simulink model "KF_Problem5"  (R2025b)
settings: Solver=FixedStepDiscrete  StartTime=0.0  StopTime=34  FixedStep=1  RelTol=1e-3
libraries: matrix_library x3, simulink x2
settings Model: Creator=xox  LastModifiedBy=xox
settings OptimizationCC: BlockReduction=off  DefaultParameterBehavior=Inlined  BufferReuse=off

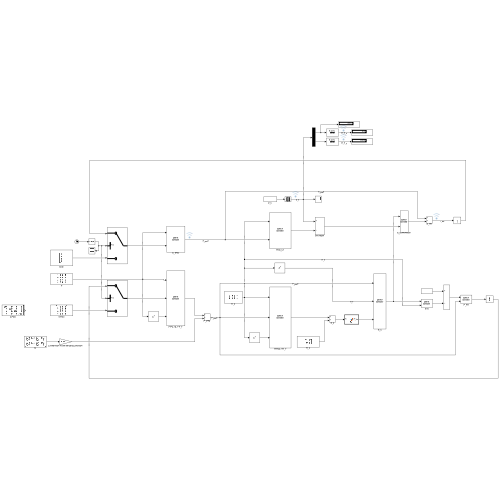
[thumbnail: Simulink's stored preview of the top-level diagram]
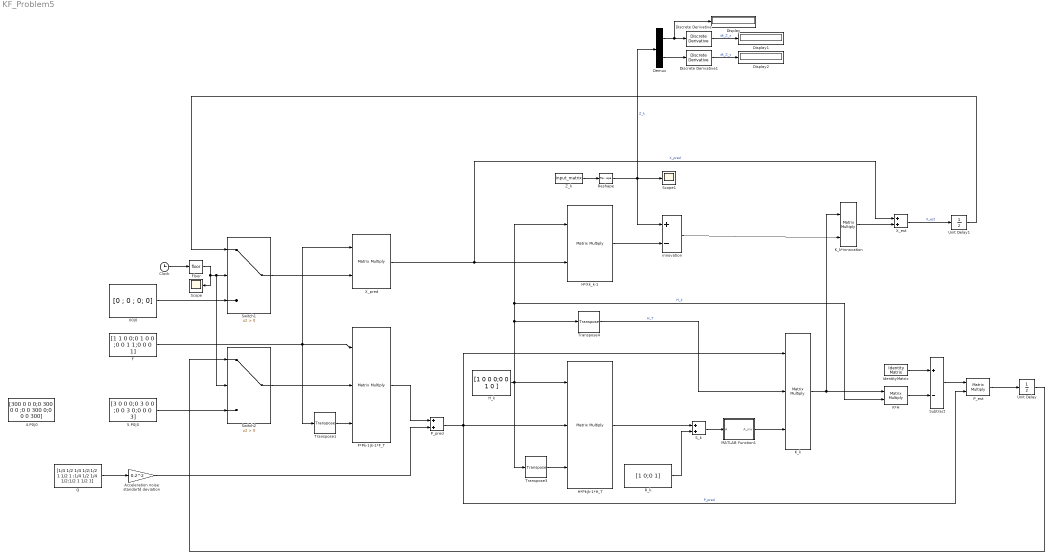
== system KF_Problem5 ==
  4.P0|0 : Constant  Value=[300 0 0 0;0 300 0 0 ;0 0 300 0;0 0 0 300]  VectorParams1D=off
  5.P0|0 : Constant  Value=[3 0 0 0;0 3 0 0 ;0 0 3 0;0 0 0 3]  VectorParams1D=off
  Acceleration noise standartd deviation : Gain  Gain=0.2^2
  Clock : Clock
  Demux : Demux  Outputs=2
  Discrete Derivative : simulink/Discrete/Discrete Derivative  gainval=1.0  ICPrevScaledInput=0.0  OutMin=[]  OutMax=[]  OutDataType=fixdt(1, 16)  OutScaling=2^-10  DoSatur=off
  Discrete Derivative1 : simulink/Discrete/Discrete Derivative  gainval=1.0  ICPrevScaledInput=0.0  OutMin=[]  OutMax=[]  OutDataType=fixdt(1, 16)  OutScaling=2^-10  DoSatur=off
  Display : Display
  Display1 : Display
  Display2 : Display
  F : Constant  Value=[1 1 0 0;0 1 0 0 ;0 0 1 1;0 0 0 1]  VectorParams1D=off
  F*Pk-1|k-1*F_T : Product  Inputs=3  Multiplication=Matrix(*)
  Floor : Rounding
  H*Pk|k-1*H_T : Product  Inputs=3  Multiplication=Matrix(*)
  H*Xk_k-1 : Product  Multiplication=Matrix(*)
  H_k : Constant  Value=[1 0 0 0;0 0 1 0 ]  VectorParams1D=off
  IdentityMatrix : IdentityMatrix  OutputDimensions=4
  K*H : Product  Multiplication=Matrix(*)
  K_k : Product  Inputs=3  Multiplication=Matrix(*)
  K_k*innovation : Product  Multiplication=Matrix(*)
  MATLAB Function1 : MATLAB Function  TreatAsAtomicUnit=on
  P_est : Product  Multiplication=Matrix(*)
  P_pred : Sum
  Q : Constant  Value=[1/4 1/2 1/4 1/2;1/2 1 1/2 1 ;1/4 1/2 1/4 1/2;1/2 1 1/2 1]  VectorParams1D=off
  R_k : Constant  Value=[1 0;0 1]  VectorParams1D=off
  Reshape : Reshape  OutputDimensionality=Column vector (2-D)
  S_k : Sum
  Scope : Scope
      settings: ActiveDisplayYMinimum=-7.79614286700194  ActiveDisplayYMaximum=47.001324962719174
  Scope1 : Scope
      settings: ActiveDisplayYMinimum=-433.90733679932936  ActiveDisplayYMaximum=356.88208874930586
  Subtract : Sum  Inputs=+-
  Switch1 : Switch  Criteria=u2 > Threshold  SaturateOnIntegerOverflow=off  InputSameDT=off
  Switch2 : Switch  Criteria=u2 > Threshold  SaturateOnIntegerOverflow=off  InputSameDT=off
  Transpose1 : matrix_library/Transpose
  Transpose3 : matrix_library/Transpose
  Transpose4 : matrix_library/Transpose
  Unit Delay : UnitDelay  SampleTime=-1  HasFrameUpgradeWarning=on
  Unit Delay1 : UnitDelay  SampleTime=-1  HasFrameUpgradeWarning=on
  X0|0 : Constant  Value=[0 ; 0 ; 0; 0]  VectorParams1D=off
  X_est : Sum
  X_pred : Product  Multiplication=Matrix(*)
  Z_k : FromWorkspace  VariableName=input_matrix
  innovation : Sum  Inputs=+-
  wires:
  Q/1 -> Acceleration noise standartd deviation/1
  S_k/1 -> MATLAB Function1/1(A)
  Clock/1 -> Floor/1
  Floor/1 -> Scope/1, Switch2/2, Switch1/2
  X0|0/1 -> Switch1/3
  F/1 -> Transpose1/1, F*Pk-1|k-1*F_T/1, X_pred/1
  Switch1/1 -> X_pred/2
  X_pred/1 -> X_est/1, H*Xk_k-1/2  "X_pred"
  Switch2/1 -> F*Pk-1|k-1*F_T/2
  Transpose1/1 -> F*Pk-1|k-1*F_T/3
  F*Pk-1|k-1*F_T/1 -> P_pred/1
  Acceleration noise standartd deviation/1 -> P_pred/2
  Z_k/1 -> Reshape/1
  Transpose3/1 -> H*Pk|k-1*H_T/3
  H_k/1 -> K*H/2, H*Xk_k-1/1, Transpose4/1, Transpose3/1, H*Pk|k-1*H_T/1  "H_k"
  P_pred/1 -> P_est/2, H*Pk|k-1*H_T/2, K_k/1  "P_pred"
  Reshape/1 -> Demux/1, innovation/1, Scope1/1  "Z_k"
  H*Xk_k-1/1 -> innovation/2
  H*Pk|k-1*H_T/1 -> S_k/1
  R_k/1 -> S_k/2
  MATLAB Function1/1(A_inv) -> K_k/3
  Transpose4/1 -> K_k/2  "H_T"
  K_k/1 -> K*H/1, K_k*innovation/1
  innovation/1 -> K_k*innovation/2
  K_k*innovation/1 -> X_est/2
  IdentityMatrix/1 -> Subtract/1
  K*H/1 -> Subtract/2
  Subtract/1 -> P_est/1
  X_est/1 -> Unit Delay1/1  "X_est"
  P_est/1 -> Unit Delay/1
  Unit Delay/1 -> Switch2/1
  Unit Delay1/1 -> Switch1/1
  Demux/1 -> Display/1, Discrete Derivative/1
  Demux/2 -> Discrete Derivative1/1
  Discrete Derivative/1 -> Display1/1  "dt_Z_x"
  Discrete Derivative1/1 -> Display2/1  "dt_Z_y"
  5.P0|0/1 -> Switch2/3

== matlab function KF_Problem5/MATLAB Function1 ==
  data: A input; A_inv output
function A_inv = fcn(A)
A_inv = inv(A);
